simulink model "prueba_doce"  (R2022b)
settings: Solver=ode4  StartTime=0  StopTime=20  FixedStep=0.0001  RelTol=1e-3
libraries: matrix_library x4
settings Model: Creator=T  LastModifiedBy=luisf
settings SolverCC: AlgebraicLoopSolver=TrustRegion
settings DataIOCC: ReturnWorkspaceOutputs=off
settings DebuggingCC: UnconnectedInputMsg=warning  UnconnectedOutputMsg=warning  UnconnectedLineMsg=warning  SFMachineParentedDataDiag=warning  ArithmeticOperatorsInVariantConditions=warning
settings ModelReferenceCC: EnableRefExpFcnMdlSchedulingChecks=on
settings SFSimCC: SimUseLocalCustomCode=off  CustomCodeUndefinedFunction=UseInterfaceOnly
settings RTWCC: RTWUseLocalCustomCode=off  DLArmComputeVersion=19.05

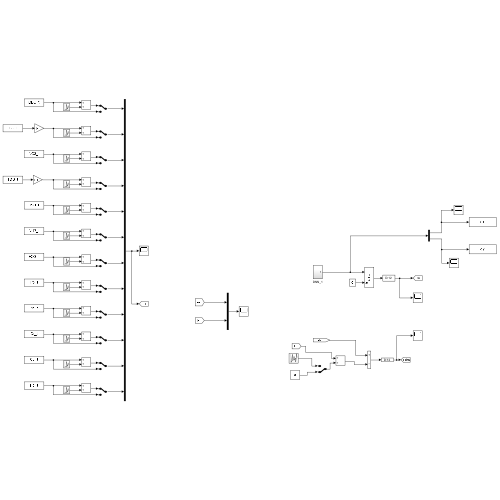
[thumbnail: Simulink's stored preview of the top-level diagram]
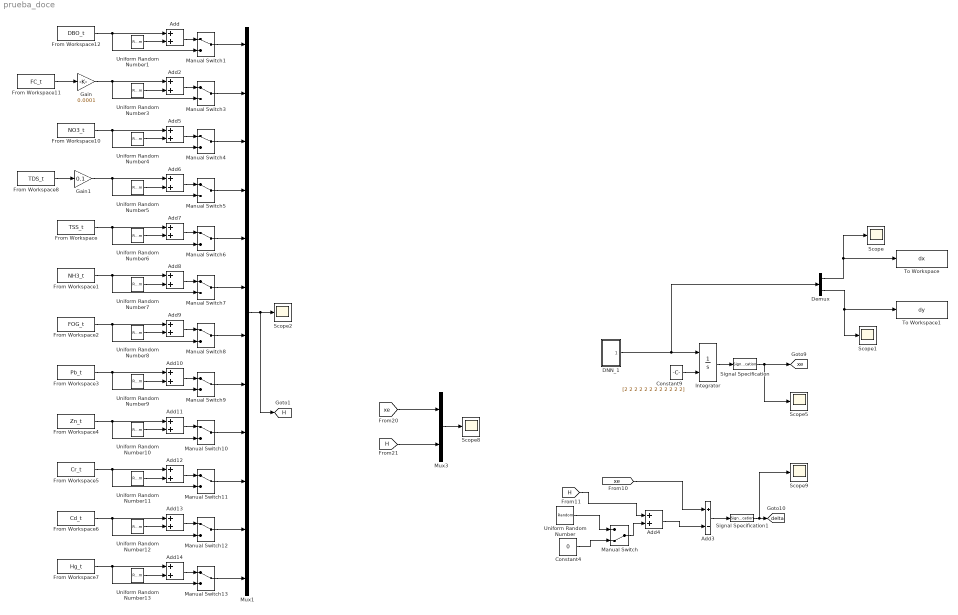
== system prueba_doce ==
  Add{,2,4..14} (13 alike) : Sum
  Add3 : Sum  Inputs=+-
  Constant4 : Constant  Value=0
  Constant9 : Constant  Value=[2 2 2 2 2 2 2 2 2 2 2 2]
  DNN_1 : Subsystem
  Demux : Demux  Outputs=2
  From Workspace : FromWorkspace  VariableName=TSS_t  SampleTime=-1
  From Workspace1 : FromWorkspace  VariableName=NH3_t  SampleTime=-1
  From Workspace10 : FromWorkspace  VariableName=NO3_t  SampleTime=-1
  From Workspace11 : FromWorkspace  VariableName=FC_t  SampleTime=-1
  From Workspace12 : FromWorkspace  VariableName=DBO_t  SampleTime=-1
  From Workspace2 : FromWorkspace  VariableName=FOG_t  SampleTime=-1
  From Workspace3 : FromWorkspace  VariableName=Pb_t  SampleTime=-1
  From Workspace4 : FromWorkspace  VariableName=Zn_t  SampleTime=-1
  From Workspace5 : FromWorkspace  VariableName=Cr_t  SampleTime=-1
  From Workspace6 : FromWorkspace  VariableName=Cd_t  SampleTime=-1
  From Workspace7 : FromWorkspace  VariableName=Hg_t  SampleTime=-1
  From Workspace8 : FromWorkspace  VariableName=TDS_t  SampleTime=-1
  Gain : Gain  Gain=0.0001
  Gain1 : Gain  Gain=0.1
  Integrator : Integrator  InitialConditionSource=external
  Manual Switch : ManualSwitch  CurrentSetting=0
  Manual Switch{1,3..13} (12 alike) : ManualSwitch
  Mux1 : Mux  Inputs=12
  Mux3 : Mux  Inputs=2
  Scope{,1..2,5,8..9} (6 alike) : Scope
  Signal Specification : SignalSpecification  Dimensions=12
  Signal Specification1 : SignalSpecification  Dimensions=12
  To Workspace : ToWorkspace  VariableName=dx  SampleTime=-1
      settings: Save2DSignal=2-D array (concatenate along first dimension)
  To Workspace1 : ToWorkspace  VariableName=dy  SampleTime=-1
      settings: Save2DSignal=2-D array (concatenate along first dimension)
  Uniform Random Number : UniformRandomNumber  Minimum=-0.01  Maximum=0.01  SampleTime=0
  Uniform Random Number1 : UniformRandomNumber  Minimum=0  Maximum=2.7  SampleTime=0.1
  Uniform Random Number10 : UniformRandomNumber  Minimum=0  Maximum=0.0064  SampleTime=0.1
  Uniform Random Number11 : UniformRandomNumber  Minimum=0  Maximum=0.0051  SampleTime=0.1
  Uniform Random Number12 : UniformRandomNumber  Minimum=0  Maximum=0.00017  SampleTime=0.1
  Uniform Random Number13 : UniformRandomNumber  Minimum=0  Maximum=0.000067  SampleTime=0.1
  Uniform Random Number3 : UniformRandomNumber  Minimum=0  Maximum=35  SampleTime=0.1
  Uniform Random Number4 : UniformRandomNumber  Minimum=0  Maximum=0.12  SampleTime=0.1
  Uniform Random Number5 : UniformRandomNumber  Minimum=0  Maximum=5.8  SampleTime=0.1
  Uniform Random Number6 : UniformRandomNumber  Minimum=0  Maximum=6.4  SampleTime=0.1
  Uniform Random Number7 : UniformRandomNumber  Minimum=0  Maximum=0.76  SampleTime=0.1
  Uniform Random Number8 : UniformRandomNumber  Minimum=0  Maximum=0.94  SampleTime=0.1
  Uniform Random Number9 : UniformRandomNumber  Minimum=0  Maximum=0.00056  SampleTime=0.1
  tag scope: H=global, delta=global, xe=global
  wires:
  Integrator/1 -> Signal Specification/1
  Constant9/1 -> Integrator/2
  Signal Specification/1 -> Scope5/1, [xe]
  Constant4/1 -> Manual Switch/2
  Uniform Random Number/1 -> Manual Switch/1
  Add3/1 -> Signal Specification1/1
  Add4/1 -> Add3/2
  [xe] -> Add3/1
  Signal Specification1/1 -> Scope9/1, [delta]
  [H] -> Add4/1
  Manual Switch/1 -> Add4/2
  Mux3/1 -> Scope8/1
  [H] -> Mux3/2
  [xe] -> Mux3/1
  DNN_1/1(Out1) -> Demux/1, Integrator/1
  Demux/2 -> Scope1/1, To Workspace1/1
  Demux/1 -> Scope/1, To Workspace/1
  Mux1/1 -> [H], Scope2/1
  From Workspace11/1 -> Gain/1
  Uniform Random Number1/1 -> Add/2
  Add/1 -> Manual Switch1/1
  Manual Switch1/1 -> Mux1/1
  From Workspace12/1 -> Manual Switch1/2, Add/1
  Gain/1 -> Manual Switch3/2, Add2/1
  Add2/1 -> Manual Switch3/1
  Uniform Random Number3/1 -> Add2/2
  Manual Switch3/1 -> Mux1/2
  From Workspace10/1 -> Manual Switch4/2, Add5/1
  Manual Switch4/1 -> Mux1/3
  Add5/1 -> Manual Switch4/1
  Uniform Random Number4/1 -> Add5/2
  Gain1/1 -> Manual Switch5/2, Add6/1
  Manual Switch5/1 -> Mux1/4
  Add6/1 -> Manual Switch5/1
  Uniform Random Number5/1 -> Add6/2
  From Workspace/1 -> Manual Switch6/2, Add7/1
  Manual Switch6/1 -> Mux1/5
  Add7/1 -> Manual Switch6/1
  Uniform Random Number6/1 -> Add7/2
  From Workspace1/1 -> Manual Switch7/2, Add8/1
  Manual Switch7/1 -> Mux1/6
  Add8/1 -> Manual Switch7/1
  Uniform Random Number7/1 -> Add8/2
  From Workspace2/1 -> Manual Switch8/2, Add9/1
  Manual Switch8/1 -> Mux1/7
  Add9/1 -> Manual Switch8/1
  Uniform Random Number8/1 -> Add9/2
  From Workspace3/1 -> Manual Switch9/2, Add10/1
  Manual Switch9/1 -> Mux1/8
  Add10/1 -> Manual Switch9/1
  Uniform Random Number9/1 -> Add10/2
  From Workspace4/1 -> Manual Switch10/2, Add11/1
  Manual Switch10/1 -> Mux1/9
  Add11/1 -> Manual Switch10/1
  Uniform Random Number10/1 -> Add11/2
  From Workspace5/1 -> Manual Switch11/2, Add12/1
  Manual Switch11/1 -> Mux1/10
  Add12/1 -> Manual Switch11/1
  Uniform Random Number11/1 -> Add12/2
  From Workspace6/1 -> Manual Switch12/2, Add13/1
  Manual Switch12/1 -> Mux1/11
  Add13/1 -> Manual Switch12/1
  Uniform Random Number12/1 -> Add13/2
  From Workspace7/1 -> Manual Switch13/2, Add14/1
  Manual Switch13/1 -> Mux1/12
  Add14/1 -> Manual Switch13/1
  Uniform Random Number13/1 -> Add14/2
  From Workspace8/1 -> Gain1/1

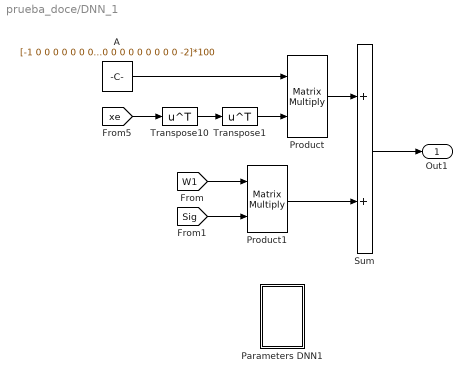
== system prueba_doce/DNN_1 ==
  A : Constant  Value=[-1 0 0 0 0 0 0 0 0 0 0 0; 0 -2 0 0 0 0 0 0 0 0 0 0; 0 0 -1 0 0 0 0 0 0 0 0 0; 0 0 0 -2 0 0 0 0 0 0 0 0; 0 0 0 0 -1 0 0 0 0 0 0 0; 0 0 0 0 0 -2 0 0 0 0 0 0; 0 0 0 0 0 0 -1 0 0 0 0 0; 0 0 0 0 0 0 0 -2 0 0 0 0; 0 0 0 0 0 0 0 0 -1 0 0 0; 0 0 0 0 0 0 0 0 0 -2 0 0; 0 0 0 0 0 0 0 0 0 0 -1 0; 0 0 0 0 0 0 0 0 0 0 0 -2]*100  VectorParams1D=off
  Parameters DNN1 : Subsystem
  Product : Product  Multiplication=Matrix(*)  SaturateOnIntegerOverflow=on  OutDataTypeStr=Inherit: Same as first input
  Product1 : Product  Multiplication=Matrix(*)  SaturateOnIntegerOverflow=on  OutDataTypeStr=Inherit: Same as first input
  Sum : Sum  SaturateOnIntegerOverflow=on
  Transpose1 : Math  Operator=transpose  SignedPower=on
  Transpose10 : Math  Operator=transpose  SignedPower=on
  Out1 : Outport  VectorParamsAs1DForOutWhenUnconnected=off
  wires:
  A/1 -> Product/1
  [W1] -> Product1/1
  [Sig] -> Product1/2
  Product/1 -> Sum/1
  Product1/1 -> Sum/2
  [xe] -> Transpose10/1
  Transpose10/1 -> Transpose1/1
  Transpose1/1 -> Product/2
  Sum/1 -> Out1/1

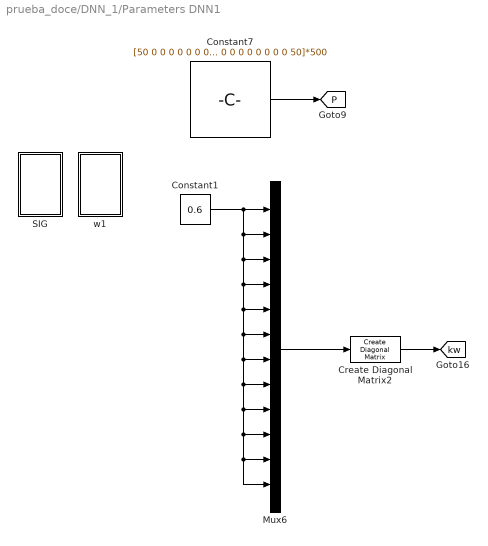
== system prueba_doce/DNN_1/Parameters DNN1 ==
  Constant1 : Constant  Value=0.6
  Constant7 : Constant  Value=[50 0 0 0 0 0 0 0 0 0 0 0; 0 50 0 0 0 0 0 0 0 0 0 0; 0 0 50 0 0 0 0 0 0 0 0 0; 0 0 0 50 0 0 0 0 0 0 0 0; 0 0 0 0 50 0 0 0 0 0 0 0; 0 0 0 0 0 50 0 0 0 0 0 0; 0 0 0 0 0 0 50 0 0 0 0 0; 0 0 0 0 0 0 0 50 0 0 0 0; 0 0 0 0 0 0 0 0 50 0 0 0; 0 0 0 0 0 0 0 0 0 50 0 0; 0 0 0 0 0 0 0 0 0 0 50 0; 0 0 0 0 0 0 0 0 0 0 0 50]*500
  Create Diagonal Matrix2 : matrix_library/Create Diagonal Matrix
  Mux6 : Mux  Inputs=12
  SIG : Subsystem
  w1 : Subsystem
  tag scope: P=global, kw=global
  wires:
  Constant7/1 -> [P]
  Create Diagonal Matrix2/1 -> [kw]
  Mux6/1 -> Create Diagonal Matrix2/1
  Constant1/1 -> Mux6/1, Mux6/2, Mux6/3, Mux6/4, Mux6/5, Mux6/6, Mux6/7, Mux6/8, Mux6/9, Mux6/10, Mux6/11, Mux6/12

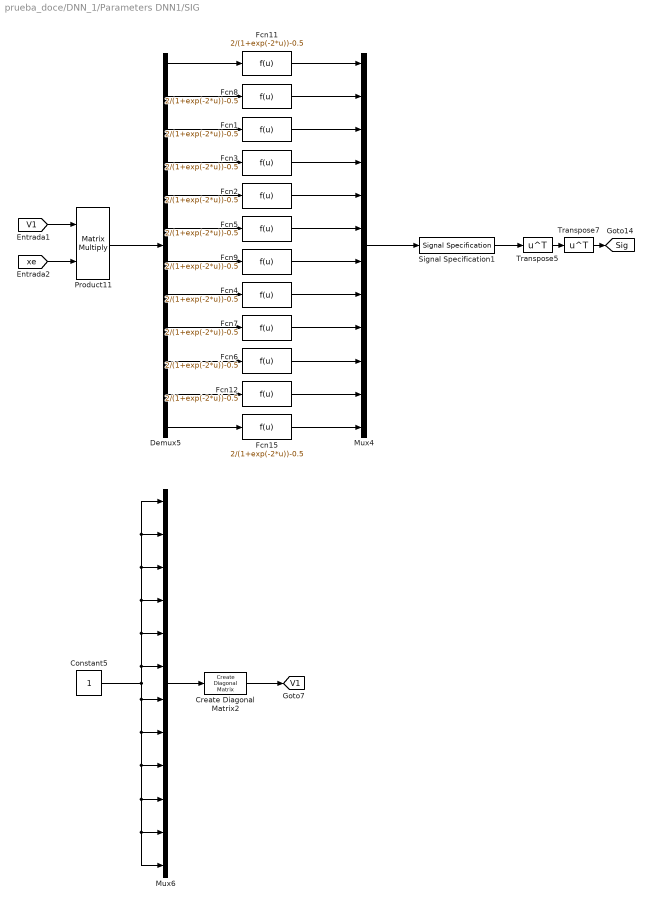
== system prueba_doce/DNN_1/Parameters DNN1/SIG ==
  Constant5 : Constant
  Create Diagonal Matrix2 : matrix_library/Create Diagonal Matrix
  Demux5 : Demux  Outputs=12
      settings: DisplayOption=none
  Fcn{1..9,11..12,15} (12 alike) : Fcn  Expr=2/(1+exp(-2*u))-0.5
  Mux4 : Mux  Inputs=12
  Mux6 : Mux  Inputs=12
  Product11 : Product  Multiplication=Matrix(*)  SaturateOnIntegerOverflow=on  OutDataTypeStr=Inherit: Same as first input
  Signal Specification1 : SignalSpecification  Dimensions=12
  Transpose5 : Math  Operator=transpose  SignedPower=on
  Transpose7 : Math  Operator=transpose  SignedPower=on
  tag scope: Sig=global, V1=global
  wires:
  Product11/1 -> Demux5/1
  [xe] -> Product11/2
  [V1] -> Product11/1
  Mux4/1 -> Signal Specification1/1
  Signal Specification1/1 -> Transpose5/1
  Transpose5/1 -> Transpose7/1
  Transpose7/1 -> [Sig]
  Create Diagonal Matrix2/1 -> [V1]
  Mux6/1 -> Create Diagonal Matrix2/1
  Constant5/1 -> Mux6/7, Mux6/8, Mux6/9, Mux6/10, Mux6/11, Mux6/12, Mux6/1, Mux6/2, Mux6/3, Mux6/4, Mux6/5, Mux6/6
  Demux5/12 -> Fcn15/1
  Fcn15/1 -> Mux4/12
  Demux5/11 -> Fcn12/1
  Fcn12/1 -> Mux4/11
  Demux5/10 -> Fcn6/1
  Demux5/9 -> Fcn7/1
  Fcn6/1 -> Mux4/10
  Fcn7/1 -> Mux4/9
  Fcn4/1 -> Mux4/8
  Demux5/8 -> Fcn4/1
  Demux5/7 -> Fcn9/1
  Fcn9/1 -> Mux4/7
  Fcn5/1 -> Mux4/6
  Demux5/6 -> Fcn5/1
  Demux5/5 -> Fcn2/1
  Fcn2/1 -> Mux4/5
  Demux5/4 -> Fcn3/1
  Fcn3/1 -> Mux4/4
  Demux5/3 -> Fcn1/1
  Demux5/2 -> Fcn8/1
  Demux5/1 -> Fcn11/1
  Fcn11/1 -> Mux4/1
  Fcn8/1 -> Mux4/2
  Fcn1/1 -> Mux4/3

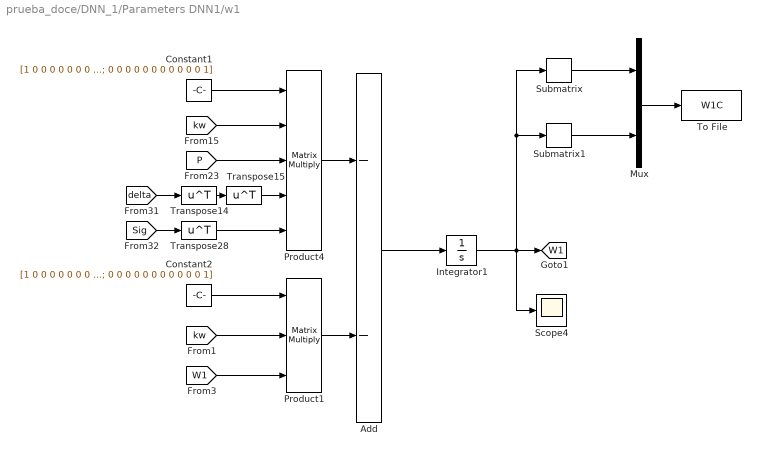
== system prueba_doce/DNN_1/Parameters DNN1/w1 ==
  Add : Sum  Inputs=--
  Constant1 : Constant  Value=[1 0 0 0 0 0 0 0 0 0 0 0; 0 1 0 0 0 0 0 0 0 0 0 0; 0 0 1 0 0 0 0 0 0 0 0 0; 0 0 0 1 0 0 0 0 0 0 0 0; 0 0 0 0 1 0 0 0 0 0 0 0; 0 0 0 0 0 1 0 0 0 0 0 0; 0 0 0 0 0 0 1 0 0 0 0 0; 0 0 0 0 0 0 0 1 0 0 0 0; 0 0 0 0 0 0 0 0 1 0 0 0; 0 0 0 0 0 0 0 0 0 1 0 0; 0 0 0 0 0 0 0 0 0 0 1 0; 0 0 0 0 0 0 0 0 0 0 0 1]
  Constant2 : Constant  Value=[1 0 0 0 0 0 0 0 0 0 0 0; 0 1 0 0 0 0 0 0 0 0 0 0; 0 0 1 0 0 0 0 0 0 0 0 0; 0 0 0 1 0 0 0 0 0 0 0 0; 0 0 0 0 1 0 0 0 0 0 0 0; 0 0 0 0 0 1 0 0 0 0 0 0; 0 0 0 0 0 0 1 0 0 0 0 0; 0 0 0 0 0 0 0 1 0 0 0 0; 0 0 0 0 0 0 0 0 1 0 0 0; 0 0 0 0 0 0 0 0 0 1 0 0; 0 0 0 0 0 0 0 0 0 0 1 0; 0 0 0 0 0 0 0 0 0 0 0 1]
  Integrator1 : Integrator  InitialCondition=[4.5 5.3 4.5 5.3 4.2 4.5 5.3 4.5 5.3 4.2 4.5 5.3; 4.5 5.3 4.5 5.3 4.2 4.5 5.3 4.5 5.3 4.2 4.5 5.3; 4.5 5.3 4.5 5.3 4.2 4.5 5.3 4.5 5.3 4.2 4.5 5.3; 4.5 5.3 4.5 5.3 4.2 4.5 5.3 4.5 5.3 4.2 4.5 5.3; 4.5 5.3 4.2 4.5 5.3 4.5 5.3 4.2 4.5 5.3 4.5 5.3; 4.5 5.3 4.2 4.5 5.3 4.5 5.3 4.2 4.5 5.3 4.5 5.3; 4.5 5.3 4.2 4.5 5.3 4.5 5.3 4.2 4.5 5.3 4.5 5.3; 4.5 5.3 4.2 4.5 5.3 4.5 5.3 4.2 4.5 5.3 4.5 5.3; 4.5 5.3 4.2 4.5 5.3 4.5 5.3 4.2 4.5 5.3 4.5 5.3; 4.5 5.3 4.2 4.5 5.3 4.5 5.3 4.2 4.5 5.3 4.5 5.3; 4.5 5.3 4.2 4.5 5.3 4.5 5.3 4.2 4.5 5.3 4.5 5.3; 4.5 5.3 4.2 4.5 5.3 4.5 5.3 4.2 4.5 5.3 4.5 5.3] *0.01  ZeroCross=off
  Mux : Mux  Inputs=2
  Product1 : Product  Inputs=3  Multiplication=Matrix(*)  SaturateOnIntegerOverflow=on  OutDataTypeStr=Inherit: Same as first input
  Product4 : Product  Inputs=5  Multiplication=Matrix(*)  SaturateOnIntegerOverflow=on  OutDataTypeStr=Inherit: Same as first input
  Scope4 : Scope
  Submatrix : matrix_library/Submatrix  RowSpan=Range of rows  RowStartMode=First  RowStartIndex=1  RowEndMode=Last  RowEndIndex=1  ColSpan=One column  ColStartMode=Index  ColStartIndex=1  ColEndMode=Last  ColEndIndex=1
  Submatrix1 : matrix_library/Submatrix  RowSpan=Range of rows  RowStartMode=First  RowStartIndex=1  RowEndMode=Last  RowEndIndex=1  ColSpan=One column  ColStartMode=Index  ColStartIndex=2  ColEndMode=Last  ColEndIndex=1
  To File : ToFile  Filename=W1C  MatrixName=W1I
  Transpose14 : Math  Operator=transpose  SignedPower=on
  Transpose15 : Math  Operator=transpose  SignedPower=on
  Transpose28 : Math  Operator=transpose  SignedPower=on
  tag scope: W1=global
  wires:
  Add/1 -> Integrator1/1
  Submatrix/1 -> Mux/1
  Submatrix1/1 -> Mux/2
  Mux/1 -> To File/1
  Integrator1/1 -> Submatrix/1, Submatrix1/1, [W1], Scope4/1
  [Sig] -> Transpose28/1
  Transpose14/1 -> Transpose15/1
  [delta] -> Transpose14/1
  [kw] -> Product1/2
  Constant2/1 -> Product1/1
  [W1] -> Product1/3
  Product4/1 -> Add/1
  Product1/1 -> Add/2
  Transpose28/1 -> Product4/5
  Transpose15/1 -> Product4/4
  [P] -> Product4/3
  [kw] -> Product4/2
  Constant1/1 -> Product4/1
